simulink model "pendule_inv_echant_etu"  (R2021a)
settings: Solver=ode45  StartTime=0.0  StopTime=100  RelTol=1e-3
values from neighbouring files (symbols this model uses):
  delta_t = 0.4    [simu_pendule_inv_echant_etu.m]
  K = [10 1]    [simu_pendule_inv_capteur_etu.m]    (also in simu_pendule_inv_echant_etu.m = [30 10]; simu_pendule_inv_etu.m = [30 10])
  ue = 0    [simu_pendule_inv_capteur_etu.m]    (also in simu_pendule_inv_echant_etu.m; simu_pendule_inv_etu.m)
  x0 = [pi/20 0]'    [simu_pendule_inv_capteur_etu.m]    (also in simu_pendule_inv_echant_etu.m; simu_pendule_inv_etu.m = [pi/10 0]')
  xe = [0 0]'    [simu_pendule_inv_capteur_etu.m]    (also in simu_pendule_inv_echant_etu.m; simu_pendule_inv_etu.m)
undefined symbols (not defined in the file or in its folder): DiscIntNeverNeededParam
settings Model: Creator=ialouane  LastModifiedBy=ialouane

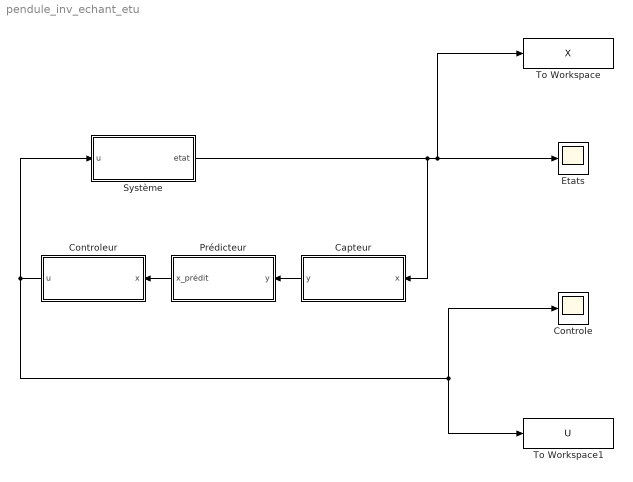
== system pendule_inv_echant_etu ==
  Capteur : Subsystem
  Controle : Scope
  Controleur : Subsystem
  Etats : Scope
  Prédicteur : Subsystem
  Système : Subsystem
  To Workspace : ToWorkspace  VariableName=X  SaveFormat=Timeseries  SampleTime=-1
  To Workspace1 : ToWorkspace  VariableName=U  SaveFormat=Timeseries  SampleTime=-1
  wires:
  Capteur/1(y) -> Prédicteur/1(y)
  Prédicteur/1(x_prédit) -> Controleur/1(x)
  Système/1(etat) -> Capteur/1(x), To Workspace/1, Etats/1
  Controleur/1(u) -> Système/1(u), To Workspace1/1, Controle/1

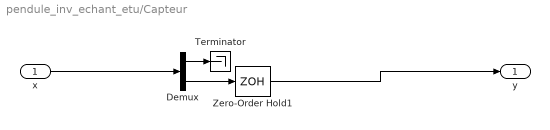
== system pendule_inv_echant_etu/Capteur ==
  x : Inport
  Demux : Demux  Outputs=2
  Terminator : Terminator
  Zero-Order Hold1 : ZeroOrderHold  SampleTime=delta_t
  y : Outport
  wires:
  Zero-Order Hold1/1 -> y/1
  Demux/2 -> Zero-Order Hold1/1
  Demux/1 -> Terminator/1
  x/1 -> Demux/1

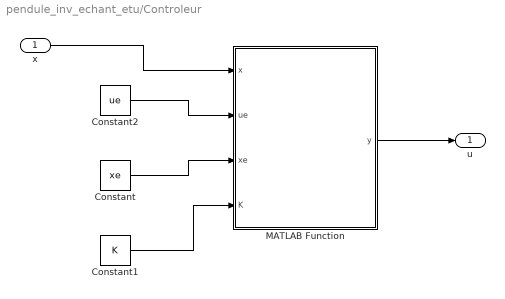
== system pendule_inv_echant_etu/Controleur ==
  x : Inport
  Constant : Constant  Value=xe
  Constant1 : Constant  Value=K  VectorParams1D=off
  Constant2 : Constant  Value=ue
  MATLAB Function : MATLAB Function  TreatAsAtomicUnit=on
  u : Outport
  wires:
  Constant2/1 -> MATLAB Function/2(ue)
  x/1 -> MATLAB Function/1(x)
  Constant/1 -> MATLAB Function/3(xe)
  Constant1/1 -> MATLAB Function/4(K)
  MATLAB Function/1(y) -> u/1

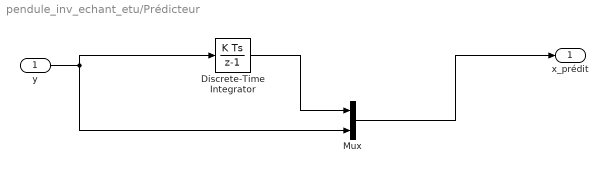
== system pendule_inv_echant_etu/Prédicteur ==
  y : Inport
  Discrete-Time Integrator : DiscreteIntegrator  InitialCondition=x0(1)  SampleTime=-1  ICPrevOutput=DiscIntNeverNeededParam  ICPrevScaledInput=DiscIntNeverNeededParam
  Mux : Mux  Inputs=2
  x_prédit : Outport
  wires:
  y/1 -> Mux/2, Discrete-Time Integrator/1
  Discrete-Time Integrator/1 -> Mux/1
  Mux/1 -> x_prédit/1

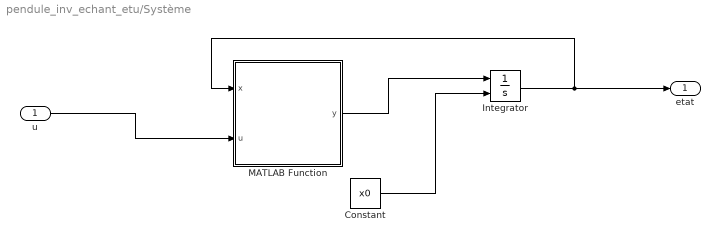
== system pendule_inv_echant_etu/Système ==
  u : Inport
  Constant : Constant  Value=x0
  Integrator : Integrator  InitialConditionSource=external
  MATLAB Function : MATLAB Function  TreatAsAtomicUnit=on
  etat : Outport
  wires:
  u/1 -> MATLAB Function/2(u)
  MATLAB Function/1(y) -> Integrator/1
  Constant/1 -> Integrator/2
  Integrator/1 -> MATLAB Function/1(x), etat/1

== matlab function pendule_inv_echant_etu/Controleur/MATLAB Function ==
  data: x input; y output; ue input; xe input; K input
function y = fcn(x,ue,xe,K)
y = ue+(K*(x-xe));

== matlab function pendule_inv_echant_etu/Système/MATLAB Function ==
  data: x input; u input; y output
function y = fcn(x,u)
l=10;
g=9.81;
y= [x(2);g/l*sin(x(1)) - cos(x(1))*u/l];
end
